simulink model "Bike"  (R2023b)
settings: Solver=FixedStepDiscrete  StartTime=0.0  StopTime=0.5  FixedStep=0.01  RelTol=1e-3
settings Model: Creator=Pranav  LastModifiedBy=Pranav

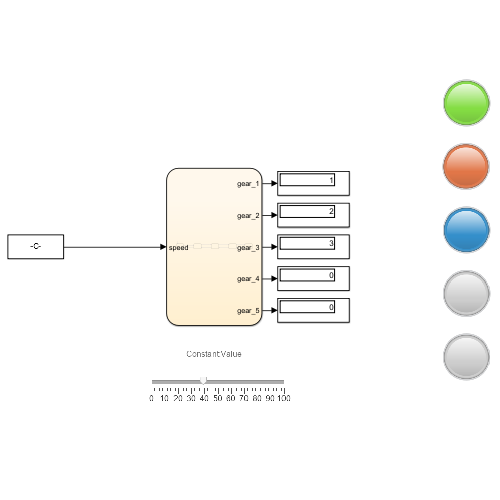
[thumbnail: Simulink's stored preview of the top-level diagram]
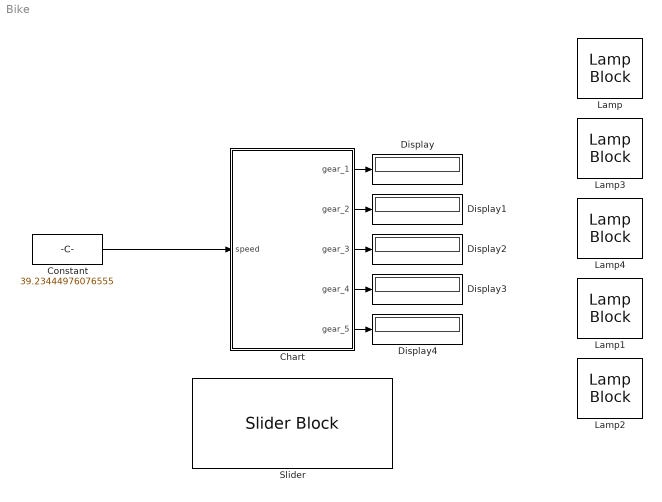
== system Bike ==
  Chart : Stateflow chart  TreatAsAtomicUnit=on
  Constant : Constant  Value=39.23444976076555
  Display{,1..4} (5 alike) : Display
  Lamp{,1..4} (5 alike) : LampBlock  LabelPosition=Hide
  Slider : SliderBlock
  wires:
  Constant/1 -> Chart/1(speed)
  Chart/1(gear_1) -> Display/1
  Chart/2(gear_2) -> Display1/1
  Chart/3(gear_3) -> Display2/1
  Chart/4(gear_4) -> Display3/1
  Chart/5(gear_5) -> Display4/1

== stateflow chart Bike/Chart ==
  state state0
    gear_1=1;
  state state1
    gear_2=2;
  state state2
    gear_3=3;
  state state3
    gear_4=4;
  state state4
    gear_5=5;
  (default) -> state0
  state1 -> state2 [order 1] : [speed>50]
  state2 -> state3 [order 1] : [speed>70]
  state3 -> state4 [order 1] : [speed>90]
  state0 -> state1 : [speed>30]
  state2 -> state1 [order 2] : [speed<50&&speed>=30]
  state4 -> state3 : [speed<90&&speed>=70]
  state3 -> state2 [order 2] : [speed<70&&speed>=50]
  state1 -> state0 [order 2] : [speed<30]
  data: speed input; gear_1 output; gear_2 output; gear_3 output; gear_4 output; gear_5 output
